simulink model "derpage8"  (R2015b)
settings: Solver=VariableStepAuto  StartTime=0.0  StopTime=(1+63)*20  RelTol=1e-3
undefined symbols (not defined in the file or in its folder): rcosine
libraries: dspstat3 x2, dspsrcs4 x1, dspsigops x1
settings Model: Creator=coltmt  LastModifiedBy=coltmt

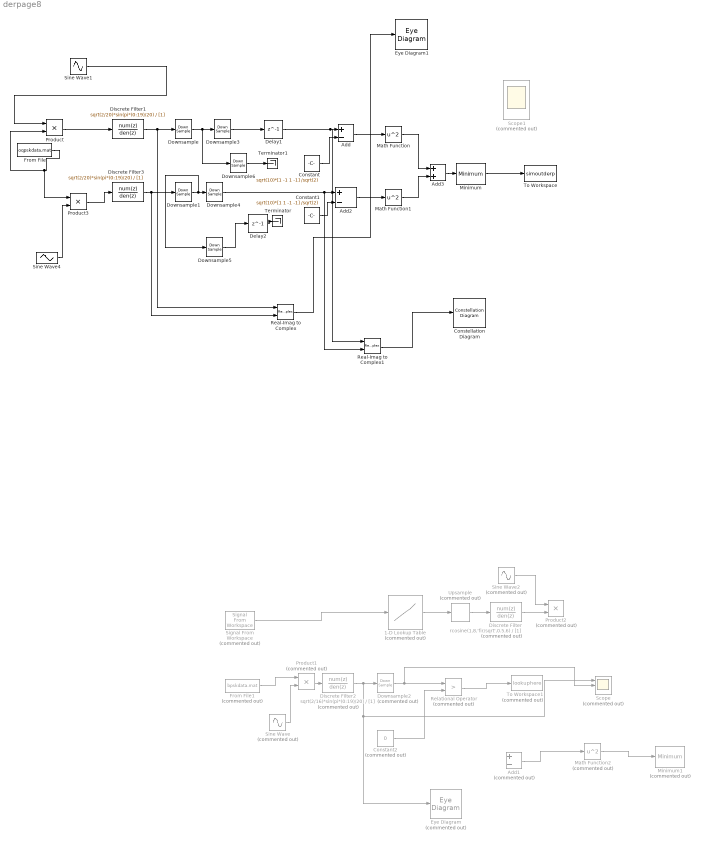
== system derpage8 ==
  1-D Lookup Table : Lookup_n-D  Commented=on  NumberOfTableDimensions=1  BreakpointsForDimension1=[0:1]  Table=[-1 1]  InternalRulePriority=Speed  RndMeth=Simplest  InputSameDT=on
  Add : Sum  Inputs=+-
  Add1 : Sum  Commented=on  Inputs=+-
  Add2 : Sum  Inputs=+-
  Add3 : Sum
  Constant : Constant  Value=sqrt(10)*[1 -1 1 -1] /sqrt(2)
  Constant1 : Constant  Value=sqrt(10)*[1 1 -1 -1] /sqrt(2)
  Constant2 : Constant  Commented=on  Value=0
  Constellation Diagram : ConstellationDiagram
  Delay1 : Delay  DelayLength=1
  Delay2 : Delay  DelayLength=1
  Discrete Filter : DiscreteFilter  Commented=on  Numerator=rcosine(1,8,'fir/sqrt',0.5,6)  Denominator=[1]
  Discrete Filter1 : DiscreteFilter  Numerator=sqrt(2/20)*sin(pi*(0:19)/20)  Denominator=[1]
  Discrete Filter2 : DiscreteFilter  Commented=on  Numerator=sqrt(2/16)*sin(pi*(0:19)/20)  Denominator=[1]
  Discrete Filter3 : DiscreteFilter  Numerator=sqrt(2/20)*sin(pi*(0:19)/20)  Denominator=[1]
  Downsample : DownSample  N=10  InputProcessing=Inherited (this choice will be removed - see release notes)  RateOptions=Allow multirate processing
  Downsample1 : DownSample  N=10  InputProcessing=Inherited (this choice will be removed - see release notes)  RateOptions=Allow multirate processing
  Downsample2 : DownSample  Commented=on  N=8  phase=1  InputProcessing=Inherited (this choice will be removed - see release notes)  RateOptions=Allow multirate processing
  Downsample3 : DownSample  RateOptions=Allow multirate processing
  Downsample4 : DownSample  phase=1  RateOptions=Allow multirate processing
  Downsample5 : DownSample  RateOptions=Allow multirate processing
  Downsample6 : DownSample  phase=1  RateOptions=Allow multirate processing
  Eye Diagram : EyeDiagram  Commented=on
  Eye Diagram1 : EyeDiagram
  From File : FromFile  FileName=oqpskdata.mat  SampleTime=1
  From File1 : FromFile  Commented=on  FileName=bpskdata.mat  OutDataTypeStr=double  SampleTime=1
  Math Function : Math  Operator=square  SaturateOnIntegerOverflow=on
  Math Function1 : Math  Operator=square  SaturateOnIntegerOverflow=on
  Math Function2 : Math  Commented=on  Operator=square  SaturateOnIntegerOverflow=on
  Minimum : dspstat3/Minimum  fcn=Index  reset=None  InputProcessing=Columns as channels (frame based)  indexBase=Zero  operateOver=Each column  Dimension=1  operation=minimum  roiEnable=off  roiType=Rectangles  roiPortion=Entire ROI  roiOutput=Individual statistics for each ROI  roiFlag=off  roundingMode=Floor  overflowMode=off
  Minimum1 : dspstat3/Minimum  Commented=on  fcn=Index  reset=None  InputProcessing=Columns as channels (frame based)  indexBase=Zero  operateOver=Each column  Dimension=1  operation=minimum  roiEnable=off  roiType=Rectangles  roiPortion=Entire ROI  roiOutput=Individual statistics for each ROI  roiFlag=off  roundingMode=Floor  overflowMode=off
  Product : Product
  Product1 : Product  Commented=on
  Product2 : Product  Commented=on
  Product3 : Product
  Real-Imag to Complex : RealImagToComplex
  Real-Imag to Complex1 : RealImagToComplex
  Relational Operator : RelationalOperator  Commented=on  Operator=>  OutDataTypeStr=boolean
  Scope : Scope  Commented=on  NumInputPorts=3
  Scope1 : Scope  Commented=on  NumInputPorts=3
  Signal From Workspace : dspsrcs4/Signal From Workspace  Commented=on  X=[1 0 0 1]  Ts=1  nsamps=1  OutputAfterFinalValue=Setting to zero  ignoreOrWarnInputAndFrameLengths=off  OutputFrames=off
  Sine Wave : Sin  Commented=on  Amplitude=sqrt(2)  Frequency=2*pi/4  Phase=pi/2  SampleTime=1
  Sine Wave1 : Sin  Amplitude=sqrt(2)  Frequency=2*pi * .3  Phase=pi/2  SampleTime=1
  Sine Wave2 : Sin  Commented=on  Amplitude=sqrt(2)  Frequency=2*pi/4  Phase=pi/2  SampleTime=1
  Sine Wave4 : Sin  Amplitude=-sqrt(2)  Frequency=2*pi * .3  SampleTime=1
  Terminator : Terminator
  Terminator1 : Terminator
  To Workspace : ToWorkspace  VariableName=simoutderp  SampleTime=-1
      settings: Save2DSignal=2-D array (concatenate along first dimension)
  To Workspace1 : ToWorkspace  Commented=on  VariableName=lookuphere  SampleTime=-1
      settings: Save2DSignal=2-D array (concatenate along first dimension)
  Upsample : dspsigops/Upsample  Commented=on  N=8  phase=0  InputProcessing=Inherited (this choice will be removed - see release notes)  RateOptions=Allow multirate processing  ic=0  mode=Unused parameter value
  wires:
  Sine Wave1/1 -> Product/1
  Sine Wave4/1 -> Product3/2
  Product/1 -> Discrete Filter1/1
  Product3/1 -> Discrete Filter3/1
  Discrete Filter3/1 -> Real-Imag to Complex/2, Downsample1/1
  Constant1/1 -> Add2/2
  Constant/1 -> Add/2
  Add/1 -> Math Function/1
  Add2/1 -> Math Function1/1
  Math Function/1 -> Add3/1
  Math Function1/1 -> Add3/2
  Add3/1 -> Minimum/1
  Minimum/1 -> To Workspace/1
  From File/1 -> Product/2, Product3/1
  Real-Imag to Complex/1 -> Eye Diagram1/1
  Real-Imag to Complex1/1 -> Constellation Diagram/1
  1-D Lookup Table/1 -> Upsample/1
  Upsample/1 -> Discrete Filter/1
  Discrete Filter2/1 -> Scope/1, Eye Diagram/1, Downsample2/1
  Downsample2/1 -> Scope/2, Relational Operator/1
  Add1/1 -> Math Function2/1
  Math Function2/1 -> Minimum1/1
  Sine Wave/1 -> Product1/2
  Product1/1 -> Discrete Filter2/1
  Discrete Filter/1 -> Product2/2
  Sine Wave2/1 -> Product2/1
  Relational Operator/1 -> To Workspace1/1
  Constant2/1 -> Relational Operator/2
  Signal From Workspace/1 -> 1-D Lookup Table/1
  From File1/1 -> Product1/1
  Downsample/1 -> Downsample6/1, Downsample3/1
  Downsample1/1 -> Downsample5/1, Downsample4/1
  Delay1/1 -> Real-Imag to Complex1/1, Add/1
  Delay2/1 -> Terminator/1
  Discrete Filter1/1 -> Real-Imag to Complex/1, Downsample/1
  Downsample4/1 -> Real-Imag to Complex1/2, Add2/1
  Downsample6/1 -> Terminator1/1
  Downsample3/1 -> Delay1/1
  Downsample5/1 -> Delay2/1
